simulink model "rocket"  (R2022b)
settings: Solver=VariableStepAuto  StartTime=0.0  StopTime=6000  RelTol=1e-3
InitFcn:
  | newrocketpara
values from neighbouring files (symbols this model uses):
  Attinit = Euler2Quat(Attinit)    [newrocketpara.m]
  Bt1 = 240    [rocketpara.m]
  Bt2 = 842    [rocketpara.m]
  Isp1s = 311.9    [rocketpara.m]
  Isp1v = 338.4    [rocketpara.m]
  Isp2 = 450.5    [rocketpara.m]
  Kp1 = 1    [newrocketpara.m]
  Kp2 = 0.5    [newrocketpara.m]
  lx1s = lx1+lx2+lx3    [newrocketpara.m]
  lx2s = lx2+lx3    [newrocketpara.m]
  lx3s = lx3    [newrocketpara.m]
  ly1 = 3.81    [rocketpara.m]
  ly2 = 3.05    [rocketpara.m]
  ly3 = 2.5    [rocketpara.m]
  Mf1 = 284089    [rocketpara.m]
  Mf2 = 20830    [rocketpara.m]
  Mp1 = Ms1+Ms2+Ms3+Mf2+Mf3    [newrocketpara.m]
  Mp2 = Ms2+Ms3+Mf3    [newrocketpara.m]
  Ms3 = 2500    [rocketpara.m]
  Msfl1 = 1256    [rocketpara.m]
  Msfl2 = 22.4465    [rocketpara.m]
  Posinit = [Rmean*cos(Lambdalatinit)*cos(Lambdaloninit);Rmean*cos(Lambdalatinit)*sin(Lambdaloninit); Rmean*sin(Lambdalatinit)]    [newrocketpara.m]
  Rmean = (a+b)/2    (= 6367444.6571)    [earthpara.m]
  Rotinit = [0;0;0]    [newrocketpara.m]
  Vinit = [0;0;0]    [newrocketpara.m]
libraries: eeGeneralControl x2
settings Model: Creator=tn  LastModifiedBy=tn
settings SolverCC: ZeroCrossAlgorithm=Adaptive
settings DataIOCC: ReturnWorkspaceOutputs=off
settings OptimizationCC: BlockReduction=off  DefaultParameterBehavior=Inlined  BufferReuse=off
settings DebuggingCC: IgnoredZcDiagnostic=none

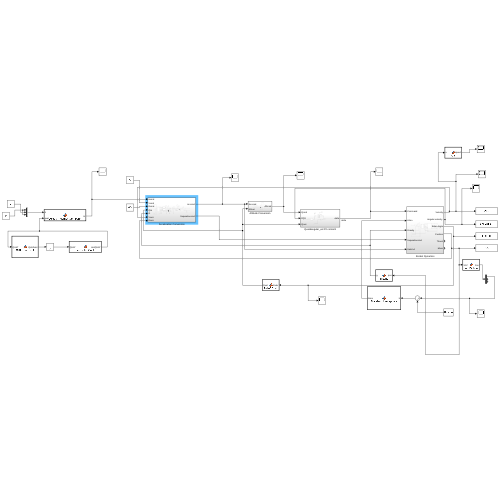
[thumbnail: Simulink's stored preview of the top-level diagram]
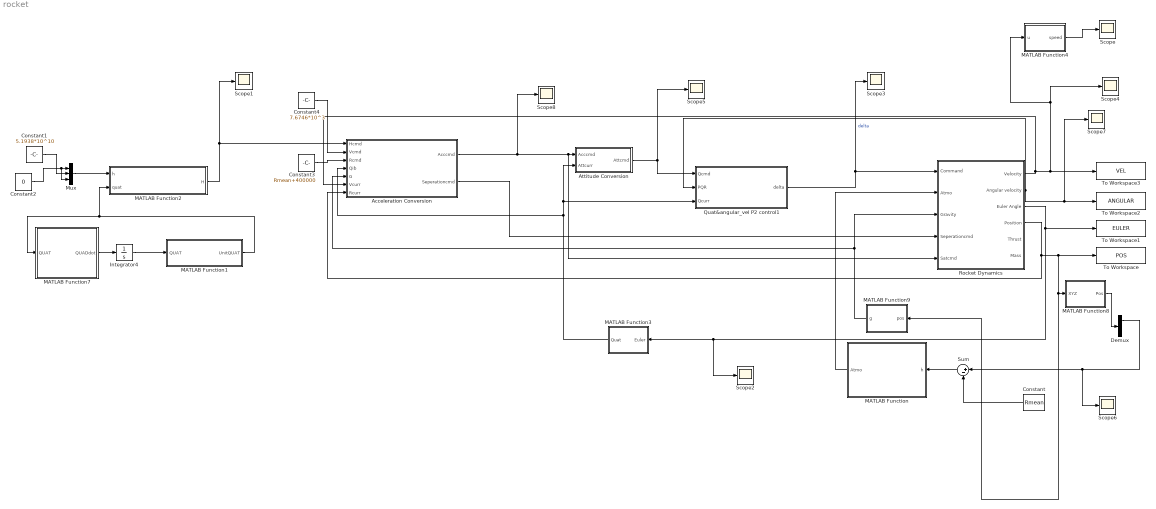
== system rocket ==
  Acceleration Conversion : Subsystem
  Attitude Conversion : Subsystem
  Constant : Constant  Value=Rmean
  Constant1 : Constant  Value=5.1938*10^10
  Constant2 : Constant  Value=0
  Constant3 : Constant  Value=Rmean+400000
  Constant4 : Constant  Value=7.6746*10^3
  Demux : Demux  Outputs=3
  Integrator4 : Integrator  InitialCondition=[1;0;0;0]
  MATLAB Function : MATLAB Function  TreatAsAtomicUnit=on
  MATLAB Function1 : MATLAB Function  TreatAsAtomicUnit=on
  MATLAB Function2 : MATLAB Function  TreatAsAtomicUnit=on
  MATLAB Function3 : MATLAB Function  TreatAsAtomicUnit=on
  MATLAB Function4 : MATLAB Function  TreatAsAtomicUnit=on
  MATLAB Function7 : MATLAB Function  TreatAsAtomicUnit=on
  MATLAB Function8 : MATLAB Function  TreatAsAtomicUnit=on
  MATLAB Function9 : MATLAB Function  TreatAsAtomicUnit=on
  Mux : Mux  Inputs=3
  Quat&angular_vel P2 control1 : Subsystem
  Rocket Dynamics : Subsystem
  Scope{,1..8} (9 alike) : Scope
  Sum : Sum  Inputs=|+-
  To Workspace : ToWorkspace  VariableName=POS  SaveFormat=Timeseries  SampleTime=-1
  To Workspace1 : ToWorkspace  VariableName=EULER  SaveFormat=Timeseries  SampleTime=-1
  To Workspace2 : ToWorkspace  VariableName=ANGULAR  SaveFormat=Timeseries  SampleTime=-1
  To Workspace3 : ToWorkspace  VariableName=VEL  SaveFormat=Timeseries  SampleTime=-1
  wires:
  Rocket Dynamics/3(Euler Angle) -> Scope2/1, MATLAB Function3/1(Euler), To Workspace1/1
  Rocket Dynamics/2("Angular velocity ") -> Scope7/1, To Workspace2/1, Quat&angular_vel P2 control1/2(PQR)
  Rocket Dynamics/1(Velocity) -> Acceleration Conversion/6(Vcurr), To Workspace3/1, MATLAB Function4/1(u), Scope4/1
  Demux/1 -> Scope6/1, Sum/1
  Constant/1 -> Sum/2
  Sum/1 -> MATLAB Function/1(h)
  MATLAB Function/1(Atmo) -> Rocket Dynamics/2(Atmo)
  MATLAB Function8/1(Pos) -> Demux/1
  MATLAB Function1/1(UnitQUAT) -> MATLAB Function2/2(quat), MATLAB Function7/1(QUAT)
  MATLAB Function7/1(QUADdot) -> Integrator4/1
  Integrator4/1 -> MATLAB Function1/1(QUAT)
  MATLAB Function3/1(Quat) -> Attitude Conversion/2(Attcurr), Quat&angular_vel P2 control1/3(Qcurr), Acceleration Conversion/4(Qib)
  Mux/1 -> MATLAB Function2/1(h)
  MATLAB Function2/1(H) -> Scope1/1, Acceleration Conversion/1(Hcmd)
  Constant3/1 -> Acceleration Conversion/3(Rcmd)
  Constant4/1 -> Acceleration Conversion/2(Vcmd)
  Quat&angular_vel P2 control1/1(delta) -> Scope3/1, Rocket Dynamics/1(Command)  "delta"
  Attitude Conversion/1(Attcmd) -> Quat&angular_vel P2 control1/1(Qcmd), Scope5/1
  Rocket Dynamics/4(Position) -> MATLAB Function9/1(pos), MATLAB Function8/1(XYZ), To Workspace/1, Acceleration Conversion/7(Rcurr)
  MATLAB Function9/1(g) -> Acceleration Conversion/5(G), Rocket Dynamics/3(Gravity)
  Constant2/1 -> Mux/3, Mux/1
  MATLAB Function4/1(speed) -> Scope/1
  Acceleration Conversion/1(Acccmd) -> Scope8/1, Rocket Dynamics/5(Satcmd), Attitude Conversion/1(Acccmd)
  Constant1/1 -> Mux/2
  Acceleration Conversion/2(Seperationcmd) -> Rocket Dynamics/4(Seperationcmd)

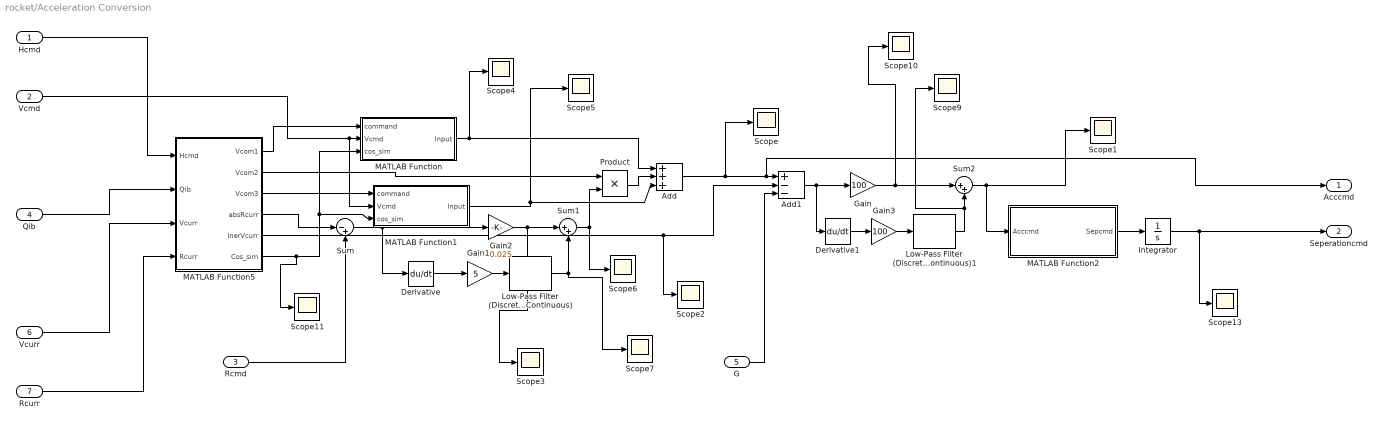
== system rocket/Acceleration Conversion ==
  Hcmd : Inport
  Vcmd : Inport  Port=2
  Rcmd : Inport  Port=3
  Qib : Inport  Port=4
  G : Inport  Port=5
  Vcurr : Inport  Port=6
  Rcurr : Inport  Port=7
  Add : Sum  Inputs=+++
  Add1 : Sum  Inputs=+--
  Derivative : Derivative  CoefficientInTFapproximation=Inf
  Derivative1 : Derivative
  Gain : Gain  Gain=100
  Gain1 : Gain  Gain=5
  Gain2 : Gain  Gain=0.025
  Gain3 : Gain  Gain=100
  Integrator : Integrator
  Low-Pass Filter (Discrete or Continuous) : eeGeneralControl/Low-Pass Filter (Discrete or Continuous)  K=1  T=1  B=inf  A=-inf  init_option=Inherited from block input  x0=0  Ts=0
  Low-Pass Filter (Discrete or Continuous)1 : eeGeneralControl/Low-Pass Filter (Discrete or Continuous)  K=1  T=10  B=inf  A=-inf  init_option=Inherited from block input  x0=0  Ts=0
  MATLAB Function : MATLAB Function  TreatAsAtomicUnit=on
  MATLAB Function1 : MATLAB Function  TreatAsAtomicUnit=on
  MATLAB Function2 : MATLAB Function  TreatAsAtomicUnit=on
  MATLAB Function5 : MATLAB Function  TreatAsAtomicUnit=on
  Product : Product
  Scope{,1..7,9..11,13} (12 alike) : Scope
  Sum : Sum  Inputs=|-+
  Sum1 : Sum  Inputs=|++
  Sum2 : Sum  Inputs=|++
  Acccmd : Outport
  Seperationcmd : Outport  Port=2
  wires:
  Hcmd/1 -> MATLAB Function5/1(Hcmd)
  Qib/1 -> MATLAB Function5/2(Qib)
  Vcurr/1 -> MATLAB Function5/3(Vcurr)
  Rcurr/1 -> MATLAB Function5/4(Rcurr)
  MATLAB Function5/1(Vcom1) -> MATLAB Function/1(command)
  MATLAB Function5/4(absRcurr) -> Sum/1
  Rcmd/1 -> Sum/2
  Sum/1 -> Gain2/1, Derivative/1
  Gain2/1 -> Scope3/1, Sum1/1
  MATLAB Function5/2(Vcom2) -> Product/1
  Sum1/1 -> Product/2, Scope6/1
  MATLAB Function5/3(Vcom3) -> MATLAB Function1/1(command)
  MATLAB Function/1(Input) -> Scope4/1, Add/1
  Product/1 -> Add/2
  MATLAB Function1/1(Input) -> Scope5/1, Add/3
  MATLAB Function5/5(InerVcurr) -> Scope2/1, Add1/2
  Add/1 -> Scope/1, Acccmd/1, Add1/1
  G/1 -> Add1/3
  Derivative/1 -> Gain1/1
  Sum2/1 -> Scope1/1, MATLAB Function2/1(Acccmd)
  Add1/1 -> Derivative1/1, Gain/1
  Vcmd/1 -> MATLAB Function1/2(Vcmd), MATLAB Function/2(Vcmd)
  MATLAB Function5/6(Cos_sim) -> Scope11/1, MATLAB Function/3(cos_sim), MATLAB Function1/3(cos_sim)
  Derivative1/1 -> Gain3/1
  Gain/1 -> Scope10/1, Sum2/1
  MATLAB Function2/1(Sepcmd) -> Integrator/1
  Integrator/1 -> Scope13/1, Seperationcmd/1
  Gain1/1 -> Low-Pass Filter (Discrete or Continuous)/1
  Low-Pass Filter (Discrete or Continuous)/1 -> Scope7/1, Sum1/2
  Gain3/1 -> Low-Pass Filter (Discrete or Continuous)1/1
  Low-Pass Filter (Discrete or Continuous)1/1 -> Scope9/1, Sum2/2

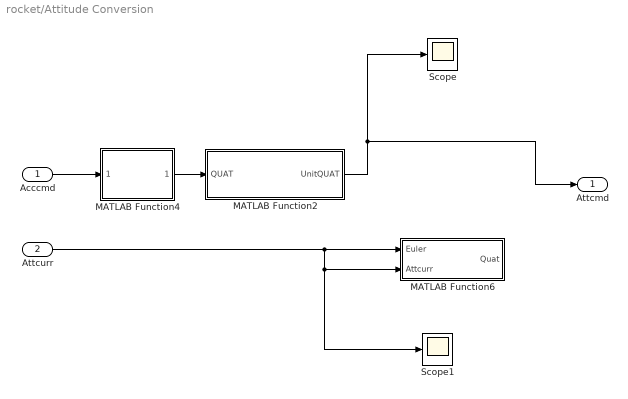
== system rocket/Attitude Conversion ==
  Acccmd : Inport
  Attcurr : Inport  Port=2
  MATLAB Function2 : MATLAB Function  TreatAsAtomicUnit=on
  MATLAB Function4 : MATLAB Function  TreatAsAtomicUnit=on
  MATLAB Function6 : MATLAB Function  TreatAsAtomicUnit=on
  Scope : Scope
  Scope1 : Scope
  Attcmd : Outport
  wires:
  Acccmd/1 -> MATLAB Function4/1(Acccmd)
  Attcurr/1 -> MATLAB Function6/1(Euler), Scope1/1, MATLAB Function6/2(Attcurr)
  MATLAB Function4/1(Attcmd) -> MATLAB Function2/1(QUAT)
  MATLAB Function2/1(UnitQUAT) -> Scope/1, Attcmd/1

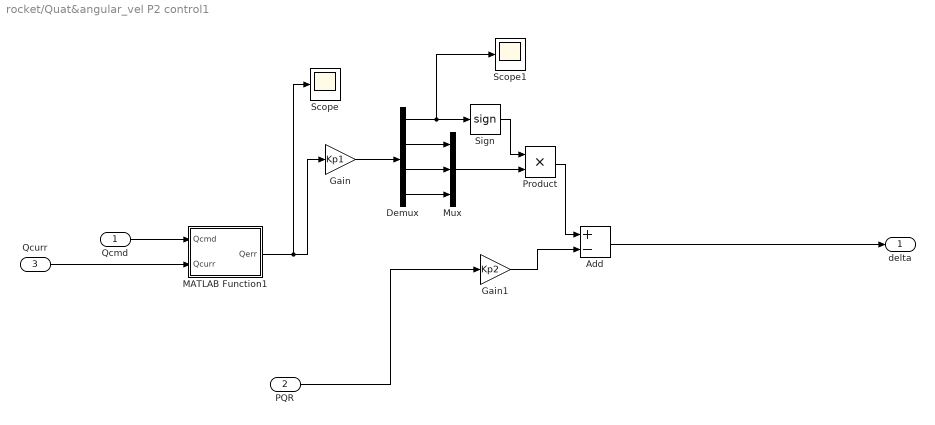
== system rocket/Quat&angular_vel P2 control1 ==
  Qcmd : Inport
  PQR : Inport  Port=2
  Qcurr : Inport  Port=3
  Add : Sum  Inputs=+-
  Demux : Demux
  Gain : Gain  Gain=Kp1
  Gain1 : Gain  Gain=Kp2
  MATLAB Function1 : MATLAB Function  TreatAsAtomicUnit=on
  Mux : Mux  Inputs=3
  Product : Product
  Scope : Scope
  Scope1 : Scope
  Sign : Signum  ZeroCross=off
  delta : Outport
  wires:
  Demux/3 -> Mux/2
  Demux/2 -> Mux/1
  MATLAB Function1/1(Qerr) -> Scope/1, Gain/1
  Gain1/1 -> Add/2
  PQR/1 -> Gain1/1
  Demux/4 -> Mux/3
  Qcurr/1 -> MATLAB Function1/2(Qcurr)
  Qcmd/1 -> MATLAB Function1/1(Qcmd)
  Gain/1 -> Demux/1
  Add/1 -> delta/1
  Demux/1 -> Scope1/1, Sign/1
  Mux/1 -> Product/2
  Sign/1 -> Product/1
  Product/1 -> Add/1

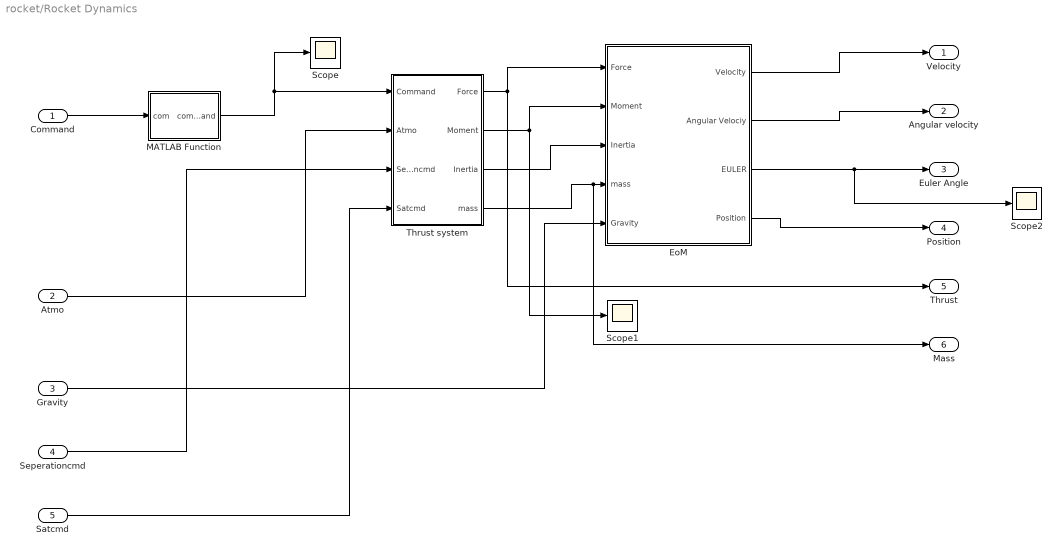
== system rocket/Rocket Dynamics ==
  Command : Inport
  Atmo : Inport  Port=2
  Gravity : Inport  Port=3
  Seperationcmd : Inport  Port=4
  Satcmd : Inport  Port=5
  EoM : Subsystem
  MATLAB Function : MATLAB Function  TreatAsAtomicUnit=on
  Scope : Scope
  Scope1 : Scope
  Scope2 : Scope
  Thrust system : Subsystem
  Velocity : Outport
  "Angular velocity " : Outport  Port=2
  Euler Angle : Outport  Port=3
  Position : Outport  Port=4
  Thrust : Outport  Port=5
  Mass : Outport  Port=6
  wires:
  Thrust system/1(Force) -> EoM/1(Force), Thrust/1
  Thrust system/2(Moment) -> Scope1/1, EoM/2(Moment)
  Thrust system/3(Inertia) -> EoM/3(Inertia)
  Thrust system/4(mass) -> Mass/1, EoM/4(mass)
  EoM/1(Velocity) -> Velocity/1
  EoM/2(Angular Velociy) -> "Angular velocity "/1
  EoM/3(EULER) -> Scope2/1, Euler Angle/1
  EoM/4(Position) -> Position/1
  Atmo/1 -> Thrust system/2(Atmo)
  Command/1 -> MATLAB Function/1(com)
  MATLAB Function/1(command) -> Scope/1, Thrust system/1(Command)
  Gravity/1 -> EoM/5(Gravity)
  Seperationcmd/1 -> Thrust system/3(Seperationcmd)
  Satcmd/1 -> Thrust system/4(Satcmd)

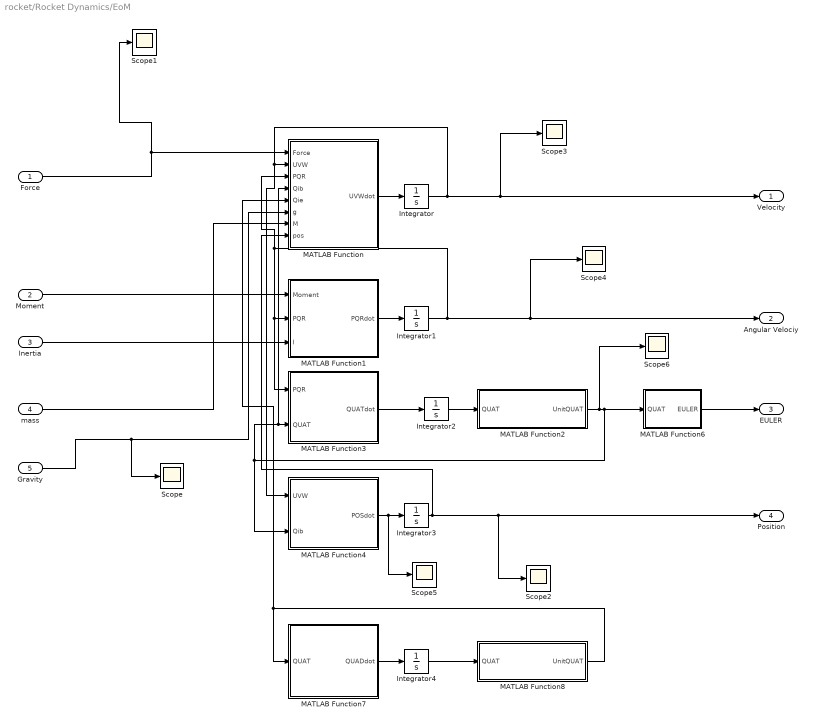
== system rocket/Rocket Dynamics/EoM ==
  Force : Inport
  Moment : Inport  Port=2
  Inertia : Inport  Port=3
  mass : Inport  Port=4
  Gravity : Inport  Port=5
  Integrator : Integrator  InitialCondition=Vinit
  Integrator1 : Integrator  InitialCondition=Rotinit
  Integrator2 : Integrator  InitialCondition=Attinit
  Integrator3 : Integrator  InitialCondition=Posinit
  Integrator4 : Integrator  InitialCondition=[1;0;0;0]
  MATLAB Function : MATLAB Function  TreatAsAtomicUnit=on
  MATLAB Function1 : MATLAB Function  TreatAsAtomicUnit=on
  MATLAB Function2 : MATLAB Function  TreatAsAtomicUnit=on
  MATLAB Function3 : MATLAB Function  TreatAsAtomicUnit=on
  MATLAB Function4 : MATLAB Function  TreatAsAtomicUnit=on
  MATLAB Function6 : MATLAB Function  TreatAsAtomicUnit=on
  MATLAB Function7 : MATLAB Function  TreatAsAtomicUnit=on
  MATLAB Function8 : MATLAB Function  TreatAsAtomicUnit=on
  Scope{,1..6} (7 alike) : Scope
  Velocity : Outport
  Angular Velociy : Outport  Port=2
  EULER : Outport  Port=3
  Position : Outport  Port=4
  wires:
  MATLAB Function2/1(UnitQUAT) -> Scope6/1, MATLAB Function6/1(QUAT), MATLAB Function4/2(Qib), MATLAB Function/4(Qib), MATLAB Function3/2(QUAT)
  Integrator1/1 -> MATLAB Function3/1(PQR), MATLAB Function1/2(PQR), MATLAB Function/3(PQR), Scope4/1, Angular Velociy/1
  MATLAB Function3/1(QUATdot) -> Integrator2/1
  MATLAB Function4/1(POSdot) -> Scope5/1, Integrator3/1
  Force/1 -> Scope1/1, MATLAB Function/1(Force)
  Integrator2/1 -> MATLAB Function2/1(QUAT)
  MATLAB Function1/1(PQRdot) -> Integrator1/1
  Integrator/1 -> Scope3/1, Velocity/1, MATLAB Function4/1(UVW), MATLAB Function/2(UVW)
  MATLAB Function6/1(EULER) -> EULER/1
  MATLAB Function/1(UVWdot) -> Integrator/1
  Moment/1 -> MATLAB Function1/1(Moment)
  Inertia/1 -> MATLAB Function1/3(I)
  mass/1 -> MATLAB Function/7(M)
  MATLAB Function7/1(QUADdot) -> Integrator4/1
  Integrator4/1 -> MATLAB Function8/1(QUAT)
  Integrator3/1 -> MATLAB Function/8(pos), Position/1, Scope2/1
  MATLAB Function8/1(UnitQUAT) -> MATLAB Function/5(Qie), MATLAB Function7/1(QUAT)
  Gravity/1 -> Scope/1, MATLAB Function/6(g)

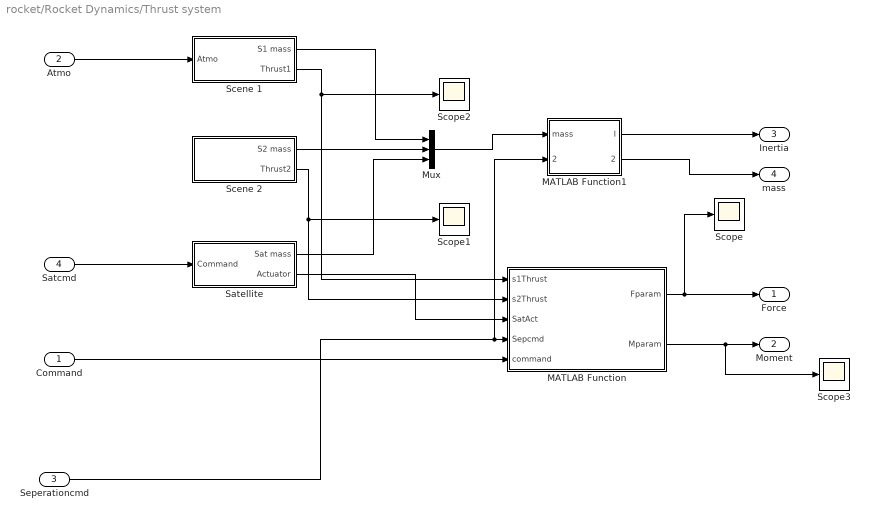
== system rocket/Rocket Dynamics/Thrust system ==
  Command : Inport
  Atmo : Inport  Port=2
  Seperationcmd : Inport  Port=3
  Satcmd : Inport  Port=4
  MATLAB Function : MATLAB Function  TreatAsAtomicUnit=on
  MATLAB Function1 : MATLAB Function  TreatAsAtomicUnit=on
  Mux : Mux  Inputs=3
  Satellite : Subsystem
  Scene 1 : Subsystem
  Scene 2 : Subsystem
  Scope{,1..3} (4 alike) : Scope
  Force : Outport
  Moment : Outport  Port=2
  Inertia : Outport  Port=3
  mass : Outport  Port=4
  wires:
  Atmo/1 -> Scene 1/1(Atmo)
  Scene 2/1(S2 mass) -> Mux/2
  Scene 1/1(S1 mass) -> Mux/1
  Satellite/1(Sat mass) -> Mux/3
  Scene 1/2(Thrust1) -> MATLAB Function/1(s1Thrust), Scope2/1
  Scene 2/2(Thrust2) -> MATLAB Function/2(s2Thrust), Scope1/1
  Satellite/2(Actuator) -> MATLAB Function/3(SatAct)
  Command/1 -> MATLAB Function/5(command)
  MATLAB Function/1(Fparam) -> Scope/1, Force/1
  Mux/1 -> MATLAB Function1/1(mass)
  MATLAB Function/2(Mparam) -> Scope3/1, Moment/1
  MATLAB Function1/1(I) -> Inertia/1
  MATLAB Function1/2(Currmass) -> mass/1
  Seperationcmd/1 -> MATLAB Function1/2(Sepcmd), MATLAB Function/4(Sepcmd)
  Satcmd/1 -> Satellite/1(Command)

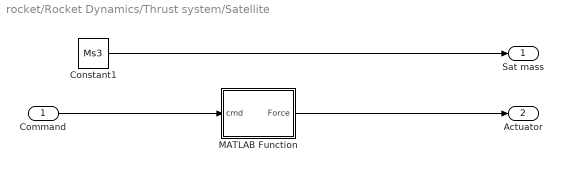
== system rocket/Rocket Dynamics/Thrust system/Satellite ==
  Command : Inport
  Constant1 : Constant  Value=Ms3
  MATLAB Function : MATLAB Function  TreatAsAtomicUnit=on
  Sat mass : Outport
  Actuator : Outport  Port=2
  wires:
  Constant1/1 -> Sat mass/1
  MATLAB Function/1(Force) -> Actuator/1
  Command/1 -> MATLAB Function/1(cmd)

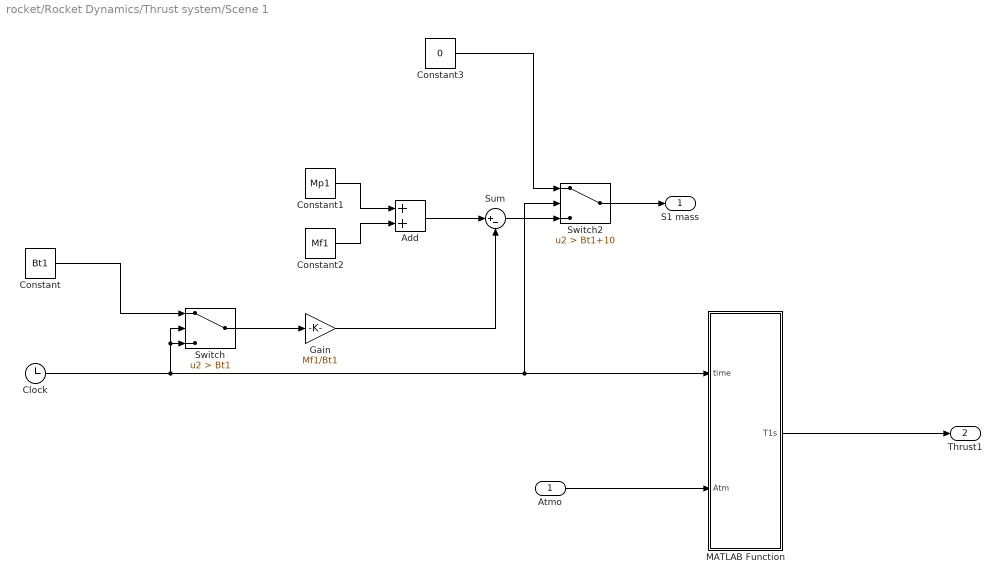
== system rocket/Rocket Dynamics/Thrust system/Scene 1 ==
  Atmo : Inport
  Add : Sum
  Clock : Clock
  Constant : Constant  Value=Bt1
  Constant1 : Constant  Value=Mp1
  Constant2 : Constant  Value=Mf1
  Constant3 : Constant  Value=0
  Gain : Gain  Gain=Mf1/Bt1
  MATLAB Function : MATLAB Function  TreatAsAtomicUnit=on
  Sum : Sum  Inputs=|+-
  Switch : Switch  Criteria=u2 > Threshold  Threshold=Bt1  SaturateOnIntegerOverflow=off  InputSameDT=off
  Switch2 : Switch  Criteria=u2 > Threshold  Threshold=Bt1+10  SaturateOnIntegerOverflow=off  InputSameDT=off
  S1 mass : Outport
  Thrust1 : Outport  Port=2
  wires:
  Clock/1 -> MATLAB Function/1(time), Switch2/2, Switch/2, Switch/3
  Constant/1 -> Switch/1
  Switch/1 -> Gain/1
  Constant1/1 -> Add/1
  Constant2/1 -> Add/2
  Add/1 -> Sum/1
  Gain/1 -> Sum/2
  Sum/1 -> Switch2/3
  Constant3/1 -> Switch2/1
  Switch2/1 -> S1 mass/1
  MATLAB Function/1(T1s) -> Thrust1/1
  Atmo/1 -> MATLAB Function/2(Atm)

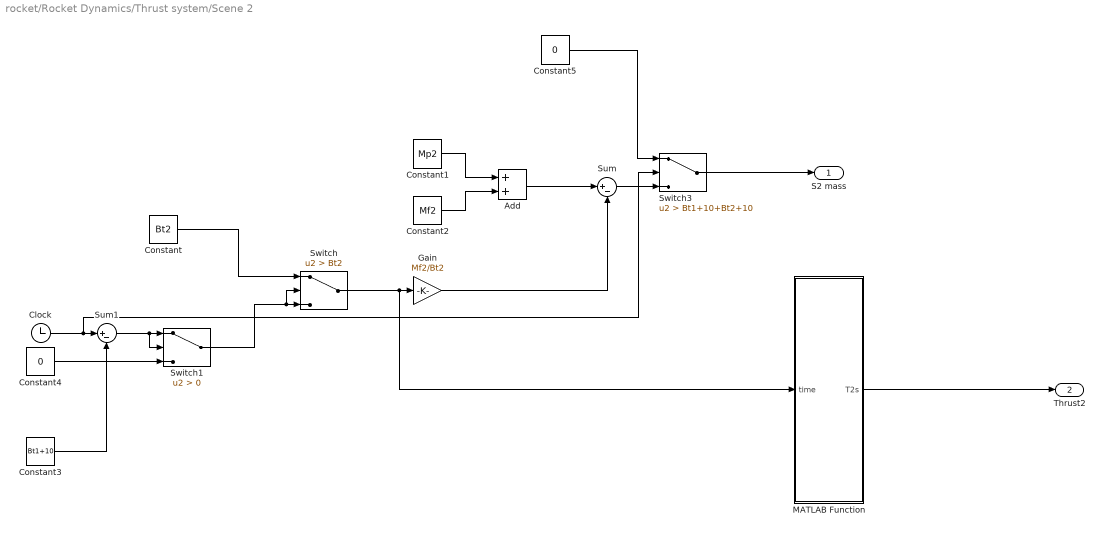
== system rocket/Rocket Dynamics/Thrust system/Scene 2 ==
  Add : Sum
  Clock : Clock
  Constant : Constant  Value=Bt2
  Constant1 : Constant  Value=Mp2
  Constant2 : Constant  Value=Mf2
  Constant3 : Constant  Value=Bt1+10
  Constant4 : Constant  Value=0
  Constant5 : Constant  Value=0
  Gain : Gain  Gain=Mf2/Bt2
  MATLAB Function : MATLAB Function  TreatAsAtomicUnit=on
  Sum : Sum  Inputs=|+-
  Sum1 : Sum  Inputs=|+-
  Switch : Switch  Criteria=u2 > Threshold  Threshold=Bt2  SaturateOnIntegerOverflow=off  InputSameDT=off
  Switch1 : Switch  Criteria=u2 > Threshold  SaturateOnIntegerOverflow=off  InputSameDT=off
  Switch3 : Switch  Criteria=u2 > Threshold  Threshold=Bt1+10+Bt2+10  SaturateOnIntegerOverflow=off  InputSameDT=off
  S2 mass : Outport
  Thrust2 : Outport  Port=2
  wires:
  Constant/1 -> Switch/1
  Switch/1 -> MATLAB Function/1(time), Gain/1
  Constant1/1 -> Add/1
  Constant2/1 -> Add/2
  Add/1 -> Sum/1
  Gain/1 -> Sum/2
  Sum/1 -> Switch3/3
  Clock/1 -> Switch3/2, Sum1/1
  Constant3/1 -> Sum1/2
  Sum1/1 -> Switch1/2, Switch1/1
  Constant4/1 -> Switch1/3
  Switch1/1 -> Switch/2, Switch/3
  Constant5/1 -> Switch3/1
  Switch3/1 -> S2 mass/1
  MATLAB Function/1(T2s) -> Thrust2/1

== matlab function rocket/Rocket Dynamics/EoM/MATLAB Function3 ==
  data: PQR input; QUAT input; QUATdot output
function QUATdot = QUAT_dot(PQR,QUAT)

q0 = QUAT(1);
q1 = QUAT(2);
q2 = QUAT(3);
q3 = QUAT(4);

p = PQR(1);
q = PQR(2);
r = PQR(3);

% q0_dot = -1/2*(q1*p +q2*q + q3*r);
% q1_dot = 1/2*(q0*p +q2*r - q3*q);
% q2_dot = 1/2*(q0*q +q3*p - q1*r);
% q3_dot = 1/2*(q0*r +q1*q - q2*p);

% QUADdot =[q0_dot; q1_dot; q2_dot; q3_dot];
QUATdot = 1/2.*Quatmul(QUAT,PQR);

== matlab function rocket/Rocket Dynamics/EoM/MATLAB Function4 ==
  data: UVW input; Qib input; POSdot output
function POSdot = POS_dot(UVW,Qib)

u = UVW(1);
v = UVW(2);
w = UVW(3);

POSdotcal = Quatmul(Quatmul(Qib,[u; v; w]), Quatinv(Qib));
POSdot = [POSdotcal(2);POSdotcal(3);POSdotcal(4)];
%POSdot = [1 0 0;0 -1 0;0 0 -1]*POSdot; % NED to ECI

== matlab function rocket/Rocket Dynamics/EoM/MATLAB Function6 ==
  data: QUAT input; EULER output
function EULER = Quat2Euler(QUAT)

q0 = QUAT(1);
q1 = QUAT(2);
q2 = QUAT(3);
q3 = QUAT(4);

phi = atan2(2*(q0*q1+q2*q3), (q0^2+q3^2-q1^2-q2^2));
theta = asin(2*(q0*q2-q1*q3));
psi = atan2(2*(q1*q2+q0*q3), (q0^2+q1^2-q2^2-q3^2));

EULER = [phi; theta; psi];

== matlab function rocket/MATLAB Function9 ==
  data: pos input; g output; mu parameter
function g = gravity(pos, mu)

x = pos(1);
y = pos(2);
z = pos(3);
r = sqrt(x^2+y^2+z^2);
normal = 1/r.*[x;y;z];

g = -mu/(r^2)*normal;

== matlab function rocket/Rocket Dynamics/EoM/MATLAB Function7 ==
  data: QUAT input; QUADdot output; wie parameter
function QUADdot = QUAT_dot_ecef(QUAT, wie)

q0 = QUAT(1);
q1 = QUAT(2);
q2 = QUAT(3);
q3 = QUAT(4);

p = 0;
q = 0;
r = wie;

q0_dot = -1/2*(q1*p +q2*q + q3*r);
q1_dot = 1/2*(q0*p +q2*r - q3*q);
q2_dot = 1/2*(q0*q +q3*p - q1*r);
q3_dot = 1/2*(q0*r +q1*q - q2*p);

QUADdot =[q0_dot; q1_dot; q2_dot; q3_dot];

== matlab function rocket/Attitude Conversion/MATLAB Function6 ==
  data: Euler input; Quat output; Attcurr input
function Quat = Euler2Quat(Euler,Attcurr)
% transformatioin from 3-2-1 rotating Euler angle rotation
if (Euler(1) > 4)
    Quat = Attcurr;
else
    phi = Euler(1);
    theta = Euler(2);
    psi = Euler(3);
    
    q0 = cos(phi/2)*cos(theta/2)*cos(psi/2) + sin(phi/2)*sin(theta/2)*sin(psi/2);
    q1 = sin(phi/2)*cos(theta/2)*cos(psi/2) - cos(phi/2)*sin(theta/2)*sin(psi/2);
    q2 = cos(phi/2)*sin(theta/2)*cos(psi/2) + sin(phi/2)*cos(theta/2)*sin(psi/2);
    q3 = cos(phi/2)*cos(theta/2)*sin(psi/2) - sin(phi/2)*sin(theta/2)*cos(psi/2);
    
    Quat = [q0;q1;q2;q3];
end
end

== matlab function rocket/Rocket Dynamics/EoM/MATLAB Function8 ==
  data: QUAT input; UnitQUAT output
function UnitQUAT = NormalizeQuat(QUAT)

q0 = QUAT(1);
q1 = QUAT(2);
q2 = QUAT(3);
q3 = QUAT(4);

Qabs = sqrt(q0^2+q1^2+q2^2+q3^2);

q0 = q0/Qabs;
q1 = q1/Qabs;
q2 = q2/Qabs;
q3 = q3/Qabs;

UnitQUAT = [q0;q1;q2;q3];
end

== matlab function rocket/MATLAB Function ==
  data: h input; Atmo output
function Atmo = Standard_Atmosphere(h)

if h < 11000
        T = 288.15 - 0.0065.*h;
        P = 101.325.*(T./288.15).^5.2559;
        rho = P./(0.2869.*T);
elseif h < 25000
        T = 216.65;
        P = 22.632.*exp(1.73-0.0001573.*h);
        rho = P./(0.2869.*T);
else
        T = 141.95 + 0.00299.*h;
        P = 2.488.*(T./216.6).^(-11.388);
        rho = P./(0.2869.*T);
end
    Atmo = [P,T,rho];
end

== matlab function rocket/MATLAB Function8 ==
  data: XYZ input; Pos output
function Pos = Cart2Sphere(XYZ)

x = XYZ(1);
y = XYZ(2);
z = XYZ(3);
rho = sqrt(x^2+y^2+z^2);
theta = acos(sqrt(x^2+y^2)/rho);
psi = acos(x/sqrt(x^2+y^2));

Pos = [rho,theta,psi];

== matlab function rocket/MATLAB Function1 ==
  data: QUAT input; UnitQUAT output
function UnitQUAT = NormalizeQuat(QUAT)

q0 = QUAT(1);
q1 = QUAT(2);
q2 = QUAT(3);
q3 = QUAT(4);

Qabs = sqrt(q0^2+q1^2+q2^2+q3^2);

q0 = q0/Qabs;
q1 = q1/Qabs;
q2 = q2/Qabs;
q3 = q3/Qabs;

UnitQUAT = [q0;q1;q2;q3];
end

== matlab function rocket/MATLAB Function7 ==
  data: QUAT input; QUADdot output; wie parameter
function QUADdot = QUAT_dot_ecef(QUAT, wie)

q0 = QUAT(1);
q1 = QUAT(2);
q2 = QUAT(3);
q3 = QUAT(4);

p = 0;
q = 0;
r = wie;

q0_dot = -1/2*(q1*p +q2*q + q3*r);
q1_dot = 1/2*(q0*p +q2*r - q3*q);
q2_dot = 1/2*(q0*q +q3*p - q1*r);
q3_dot = 1/2*(q0*r +q1*q - q2*p);

QUADdot =[q0_dot; q1_dot; q2_dot; q3_dot];

== matlab function rocket/Rocket Dynamics/Thrust system/Scene 1/MATLAB Function ==
  data: time input; Atm input; T1s output; Isp1s parameter; Isp1v parameter; Msfl1 parameter; Bt1 parameter
function T1s = Thrust(time, Atm, Isp1s, Isp1v, Msfl1, Bt1)
if time >= Bt1
    T1s = 0;
    return
end
Const = (Isp1v - Isp1s)/(101.325);
Ispcurr = Isp1s + Const * (101.325 - Atm(1));
T1s = Msfl1*9.81*Ispcurr;

== matlab function rocket/MATLAB Function2 ==
  data: h input; H output; quat input
function H = Angular_Momentum_ECEF(h,quat)

hcal = Quatmul(Quatmul(quat,h),Quatinv(quat));

H = [hcal(2);hcal(3);hcal(4)];
H = (1/norm(H)).*H;

== matlab function rocket/MATLAB Function3 ==
  data: Euler input; Quat output
function Quat = Euler2Quat(Euler)
% transformatioin from 3-2-1 rotating Euler angle rotation

phi = Euler(1);
theta = Euler(2);
psi = Euler(3);

q0 = cos(phi/2)*cos(theta/2)*cos(psi/2) + sin(phi/2)*sin(theta/2)*sin(psi/2);
q1 = sin(phi/2)*cos(theta/2)*cos(psi/2) - cos(phi/2)*sin(theta/2)*sin(psi/2);
q2 = cos(phi/2)*sin(theta/2)*cos(psi/2) + sin(phi/2)*cos(theta/2)*sin(psi/2);
q3 = cos(phi/2)*cos(theta/2)*sin(psi/2) - sin(phi/2)*sin(theta/2)*cos(psi/2);

Quat = [q0;q1;q2;q3];
end

== matlab function rocket/Acceleration Conversion/MATLAB Function ==
  data: command input; Input output; Vcmd input; cos_sim input
function Input = gain(command, Vcmd, cos_sim)

Input = Vcmd.*abs(cos_sim).*command;

== matlab function rocket/MATLAB Function4 ==
  data: u input; speed output
function speed = fcn(u)

speed = norm(u);

== matlab function rocket/Rocket Dynamics/MATLAB Function ==
  data: com input; command output
function command = Actuator_Limit(com)

y = com(2);
z = com(3);

if (sqrt(y^2+z^2) > sind(8))
    y = sind(8)*(y/sqrt(y^2+z^2));
    z = sind(8)*(z/sqrt(y^2+z^2));
end
x = sqrt(1-(y^2+z^2));
command = [x,y,z];

== matlab function rocket/Acceleration Conversion/MATLAB Function5 ==
  data: Vcom1 output; Vcom2 output; Vcom3 output; Hcmd input; absRcurr output; Qib input; Vcurr input; Rcurr input; InerVcurr output; Cos_sim output
function [Vcom1, Vcom2, Vcom3, absRcurr, InerVcurr, Cos_sim]= Velcom(Hcmd, Qib, Vcurr, Rcurr)

% Rcmd = abs value of Rcmd vector
% Vcmd = abs value of Vcmd vector
% Rcurr = Current R vector @ inertia frame
% Vcurr = Current R vector @ body frame
absRcurr = norm(Rcurr);
normRcurr = Rcurr./absRcurr;

inerVcurr = Quatmul(Quatmul(Qib,Vcurr),Quatinv(Qib));
InerVcurr = [inerVcurr(2);inerVcurr(3);inerVcurr(4)];
% 1st velocity component
% velocity to set current radius normal to Hcmd plane
temp = ((Hcmd'*normRcurr).*Hcmd);
Cos_sim = (Hcmd'*normRcurr);
Vcom1 = -(temp-(temp'*normRcurr).*normRcurr);

% 2nd velocity component
% velocity to go commanded radius
Vcom2 = normRcurr;

% 3rd velocity component
% velocity to have commanded angular momentum
Vcom3 = cross(normRcurr, Hcmd);
if (norm(Vcom3)~=0)
    Vcom3 = Vcom3./norm(Vcom3);
else
    Vcom3 = Vcom3;
end

== matlab function rocket/Acceleration Conversion/MATLAB Function1 ==
  data: command input; Input output; Vcmd input; cos_sim input
function Input = gain(command, Vcmd, cos_sim)

Input = Vcmd.*(1-abs(cos_sim)).*command;

== matlab function rocket/Attitude Conversion/MATLAB Function4 ==
  data: Acccmd input; Attcmd output
function Attcmd = Acc2Att(Acccmd)

if (nnz(Acccmd./norm(Acccmd) == -[1;0;0]) == 3)
    Attcmd = [0;0;1;0];
    return
end

temp = cross(Acccmd,[1;0;0]);
q0 = norm(Acccmd)+dot(Acccmd,[1;0;0]);

Attcmd = [q0;temp(1);temp(2);temp(3)];
end

== matlab function rocket/Acceleration Conversion/MATLAB Function2 ==
  data: Acccmd input; Sepcmd output
function Sepcmd = SepThrcmd(Acccmd)
% Early stage seperation command for steady Velocity

MaxThr = 99200;
if (norm(Acccmd) < MaxThr*0.1)
    Sepcmd = 1;
else
    Sepcmd = 0;
end

== matlab function rocket/Rocket Dynamics/Thrust system/Satellite/MATLAB Function ==
  data: cmd input; Force output
function Force = SatSat(cmd)

normal = cmd./norm(cmd);
Force = 900*normal;

== matlab function rocket/Attitude Conversion/MATLAB Function2 ==
  data: QUAT input; UnitQUAT output
function UnitQUAT = NormalizeQuat(QUAT)

q0 = QUAT(1);
q1 = QUAT(2);
q2 = QUAT(3);
q3 = QUAT(4);

Qabs = sqrt(q0^2+q1^2+q2^2+q3^2);

q0 = q0/Qabs;
q1 = q1/Qabs;
q2 = q2/Qabs;
q3 = q3/Qabs;

UnitQUAT = [q0;q1;q2;q3];
end

== matlab function rocket/Rocket Dynamics/Thrust system/MATLAB Function1 ==
  data: mass input; Sepcmd input; I output; lx1s parameter; lx2s parameter; lx3s parameter; ly1 parameter; ly2 parameter; ly3 parameter; Currmass output
function [I, Currmass]= Inertia(mass,Sepcmd, lx1s, lx2s, lx3s, ly1, ly2, ly3)

if (Sepcmd)
    Currmass = mass(3);
    Currlx = lx3s;
    Currly = ly3;
elseif (mass(1)~=0)
    Currmass = mass(1);
    Currlx = lx1s;
    Currly = ly1;
elseif (mass(2)~=0)
    Currmass = mass(2);
    Currlx = lx2s;
    Currly = ly2;
else
    Currmass = mass(3);
    Currlx = lx3s;
    Currly = ly3;
end
Ixx = 1/2*Currmass*(Currly/2)^2;
Iyy = 1/12*Currmass*(3*(Currly/2)^2+(Currlx)^2);
Izz = Iyy;
I = [Ixx;Iyy;Izz];

== matlab function rocket/Quat&angular_vel P2 control1/MATLAB Function1 ==
  data: Qcmd input; Qerr output; Qcurr input
function Qerr = ErrorQ(Qcmd, Qcurr)

qx = Quatinv(Qcurr);

Qerr = Quatmul(qx, Qcmd);
end

== matlab function rocket/Rocket Dynamics/EoM/MATLAB Function ==
  data: Force input; UVWdot output; UVW input; PQR input; Qib input; Qie input; g input; M input; pos input; wie parameter
function UVWdot= UVW_dot(Force,UVW,PQR,Qib, Qie, g, M, pos, wie)

fx = Force(1);
fy = Force(2);
fz = Force(3);
fm = [fx;fy;fz];

u = UVW(1);
v = UVW(2);
w = UVW(3);
velm = [u;v;w];

p = PQR(1);
q = PQR(2);
r = PQR(3);

x=pos(1);
y=pos(2);
z=pos(3);
posm = Quatmul(Quatmul(Quatinv(Qib),[x;y;z]),Qib);
posm = [posm(2);posm(3);posm(4)];

gcal = Quatmul(Quatmul(Quatinv(Qib),g), Qib);
gb = [gcal(2);gcal(3);gcal(4)];
wiee = Quatmul(Quatmul(Quatinv(Qib),[0;0;wie]),Qib);
wiee = [wiee(2);wiee(3);wiee(4)];

%u_dot = v*r - w*q + fx/M + gb(1);
%v_dot = -u*r + w*p + fy/M + gb(2);
%w_dot = u*q - v*p + fz/M + gb(3);

UVWdot =1/M.*fm+gb-cross(PQR-wiee,UVW)-2.*cross(wiee,UVW)-cross(wiee,cross(wiee,posm));

== matlab function rocket/Rocket Dynamics/Thrust system/Scene 2/MATLAB Function ==
  data: time input; Msfl2 parameter; T2s output; Bt2 parameter; Isp2 parameter
function T2s = Thrust(time, Msfl2, Bt2, Isp2)
if (time >= Bt2 || time ==0)
    T2s = 0;
    return
end

T2s = Msfl2*9.81*Isp2;

== matlab function rocket/Rocket Dynamics/EoM/MATLAB Function1 ==
  data: Moment input; PQRdot output; PQR input; I input
function PQRdot = PQR_dot(Moment, PQR, I)

Ixx = I(1);
Iyy = I(2);
Izz = I(3);
p = PQR(1);
q = PQR(2);
r = PQR(3);

% L=0, So p_dot is zero, p is constant value
L = Moment(1);
M = Moment(2);
N = Moment(3);

p_dot = L/Ixx - (Izz-Iyy)*q*r/Ixx;
q_dot = M/Iyy - (Ixx-Izz)*p*r/Iyy;
r_dot = N/Izz - (Iyy-Ixx)*p*q/Izz;

PQRdot = [p_dot;q_dot;r_dot];

== matlab function rocket/Rocket Dynamics/EoM/MATLAB Function2 ==
  data: QUAT input; UnitQUAT output
function UnitQUAT = NormalizeQuat(QUAT)

q0 = QUAT(1);
q1 = QUAT(2);
q2 = QUAT(3);
q3 = QUAT(4);

Qabs = sqrt(q0^2+q1^2+q2^2+q3^2);

q0 = q0/Qabs;
q1 = q1/Qabs;
q2 = q2/Qabs;
q3 = q3/Qabs;

UnitQUAT = [q0;q1;q2;q3];
end

== matlab function rocket/Rocket Dynamics/Thrust system/MATLAB Function ==
  data: s1Thrust input; Fparam output; s2Thrust input; SatAct input; Sepcmd input; command input; lx1s parameter; lx2s parameter; Mparam output
function [Fparam, Mparam]= TotalThrust(s1Thrust, s2Thrust, SatAct, Sepcmd, command, lx1s, lx2s)

if (Sepcmd)
    Fparam = SatAct(1:3);
    Mparam = [0;0;0];
    return
end
if (s1Thrust~=0)
    CurrThrust = s1Thrust;
    CurrArm = lx1s/2;
elseif (s2Thrust~=0)
    CurrThrust = s2Thrust;
    CurrArm = lx2s/2;
else
    Fparam = SatAct(1:3);
    Mparam = [0;0;0];
    return

end
    Fparam = CurrThrust*[command(1);-command(3);command(2)];
    Mparam = CurrThrust*[0;CurrArm*command(2);CurrArm*command(3)];
